simulink model "TVC_Rocket_Model"  (R2025b)
settings: Solver=VariableStepAuto  StartTime=0.0  StopTime=10  RelTol=1e-6
PostLoadFcn:
  | VSS_MODE = 0;
model workspace (MAT data in the model file):
  MMI = 0.012155
  TVC_max = 0.087
  moment_arm = 0.2
  thrust = 14.3
undefined symbols (not defined in the file): Kd, Kp, slew, tau_sensor, theta0
libraries: simulink x1, slpidlib x1, shared3dof x1
settings Model: Creator=joebarnard  LastModifiedBy=braxt
settings SolverCC: ZeroCrossAlgorithm=Adaptive
settings DataIOCC: Refine=5
settings DebuggingCC: IgnoredZcDiagnostic=none  UnconnectedInputMsg=warning  UnconnectedOutputMsg=warning  UnconnectedLineMsg=warning
settings ModelReferenceCC: EnableRefExpFcnMdlSchedulingChecks=on
settings RTWCC: GPUComputeCapability=3.5  DLArmComputeVersion=19.05

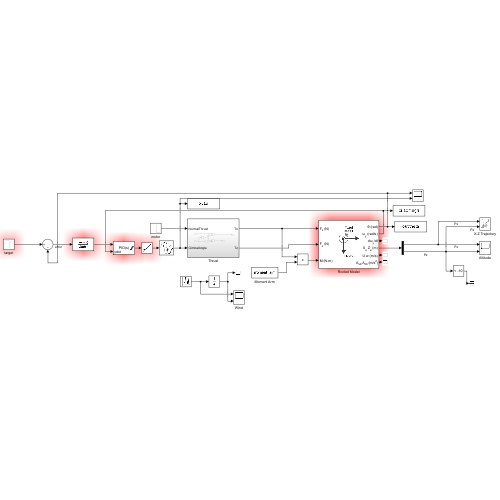
[thumbnail: Simulink's stored preview of the top-level diagram]
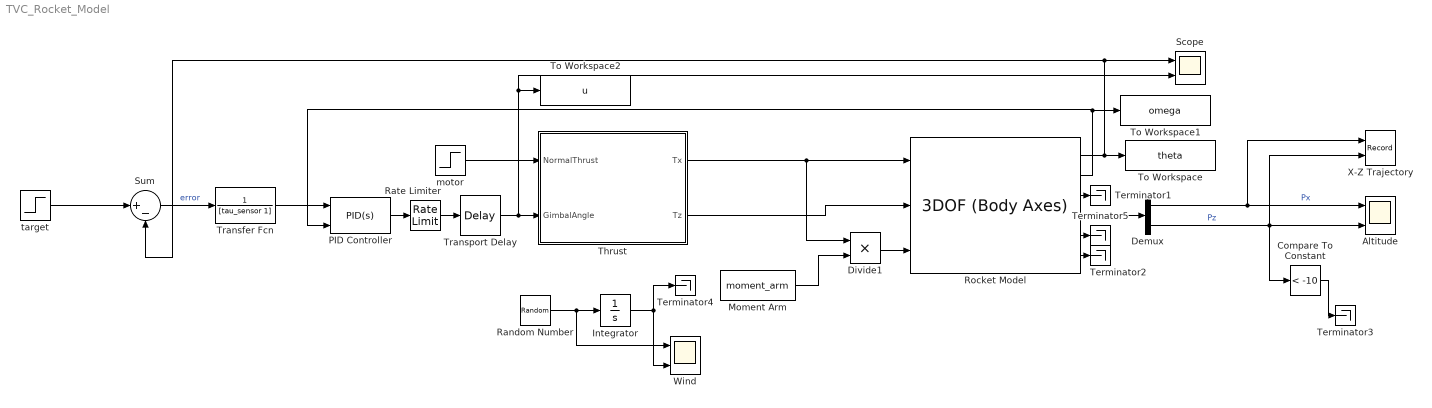
== system TVC_Rocket_Model ==
  Altitude : Scope  NumInputPorts=2
      settings: ActiveDisplayYMinimum=-149.51861  ActiveDisplayYMaximum=1345.66746  DataLoggingVariableName=ScopeData2
  Compare To Constant : simulink/Logic and Bit Operations/Compare To Constant  relop=<  const=-10  OutDataTypeStr=boolean
  Demux : Demux  Outputs=2
  Divide1 : Product  Inputs=**
  Integrator : Integrator
  "Moment Arm " : Constant  Value=moment_arm
  PID Controller : slpidlib/PID Controller  Controller=PID  Form=Parallel  TimeDomain=Continuous-time  UseExternalTs=off  SampleTime=-1  IntegratorMethod=Forward Euler  FilterMethod=Forward Euler  ControllerParametersSource=internal  P=Kp  I=0  UseKiTs=off  D=Kd  UseExternalDerivativeSource=on  N=100  UseFilter=on  TunerSelectOption=Transfer Function Based (PID Tuner App)  InitialConditionSource=internal  InitialConditionForIntegrator=0  InitialConditionForFilter=0  DifferentiatorICPrevScaledInput=0  ExternalReset=none  TrackingMode=off  Kt=1  LimitOutput=on  SatLimitsSource=internal  UpperSaturationLimit=0.087  LowerSaturationLimit=-0.087  LinearizeAsGain=on  AntiWindupMode=none  Kb=1  LimitIntegrator=off  UpperIntegratorSaturationLimit=inf  LowerIntegratorSaturationLimit=-inf  POutMin=[]  POutMax=[]  IOutMin=[]  IOutMax=[]  DOutMin=[]  DOutMax=[]  NOutMin=[]  NOutMax=[]  SumOutMin=[]  SumOutMax=[]  SaturationOutMin=[]  SaturationOutMax=[]  PParamMin=[]  PParamMax=[]  IParamMin=[]  IParamMax=[]  DParamMin=[]  DParamMax=[]  NParamMin=[]  NParamMax=[]  KbParamMin=[]  KbParamMax=[]  KtParamMin=[]  KtParamMax=[]  KbOutMin=[]  KbOutMax=[]  KtOutMin=[]  KtOutMax=[]  IntegratorOutMin=[]  IntegratorOutMax=[]  FilterOutMin=[]  FilterOutMax=[]  SumI1OutMin=[]  SumI1OutMax=[]  SumI2OutMin=[]  SumI2OutMax=[]  SumI3OutMin=[]  SumI3OutMax=[]  SumI4OutMin=[]  SumI4OutMax=[]  SumDOutMin=[]  SumDOutMax=[]  DifferentiatorOutMin=[]  DifferentiatorOutMax=[]  FilterDiffOutCoefMin=[]  FilterDiffOutCoefMax=[]  ReciprocalOutMin=[]  ReciprocalOutMax=[]  SumDenOutMin=[]  SumDenOutMax=[]  SumNumOutMin=[]  SumNumOutMax=[]  DivideOutMin=[]  DivideOutMax=[]  UdiffTsProdOutMin=[]  UdiffTsProdOutMax=[]  NTsProdOutMin=[]  NTsProdOutMax=[]  UintegralTsProdOutMin=[]  UintegralTsProdOutMax=[]  UngainTsProdOutMin=[]  UngainTsProdOutMax=[]  ClampingZeroOutDataTypeStr=Inherit: Inherit via back propagation  ClampingZeroOutMin=[]  ClampingZeroOutMax=[]  FilterDenConstantOutDataTypeStr=Inherit: Inherit via back propagation  FilterDenConstantOutMin=[]  FilterDenConstantOutMax=[]  PCopyOutDataTypeStr=Inherit: Inherit via back propagation  PCopyOutMin=[]  PCopyOutMax=[]  NCopyOutDataTypeStr=Inherit: Inherit via back propagation  NCopyOutMin=[]  NCopyOutMax=[]  IntegratorContinuousStateAttributes=''  IntegratorStateMustResolveToSignalObject=off  IntegratorRTWStateStorageClass=Auto  FilterContinuousStateAttributes=''  FilterStateMustResolveToSignalObject=off  FilterRTWStateStorageClass=Auto  ParallelPVariant=InternalParameters  IdealPVariant=Disabled  IVariant=InternalParameters  DVariant=InternalParameters  IntegratorVariant=Continuous  SatVariant=Enabled  AWVariant=Passthrough  PCopyVariant=Disabled  TRVariant=Disabled  FdbkBlocksVariant=Forward  IdealPFdbkVariant=Disabled  SatFdbkVariant=Disabled  DerivativeFilterVariant=ContFilterOnly  NVariant=InternalParameters  NCopyVariant=Disabled  FilterICVariant=InternalICsFilter  IntegratorICVariant=InternalICs  ExternalResetVariant=Disabled  TRSumVariant=Passthrough  SumFdbkVariant=Disabled  SumVariant=Sum_PID  TsampFilterVariant=InternalTs  TsampNgainVariant=Passthrough  TsampIntegralVariant=Disabled_SignalSpec  ExternalSaturationOutDataTypeStr=Inherit: Same as second input  DerivativeSourceVariant=ExternalYdot  PreIntVariant=InternalPreInt
  Random Number : RandomNumber  Variance=0.0001  Seed=2  SampleTime=3
  Rate Limiter : RateLimiter  RisingSlewLimit=slew  FallingSlewLimit=-slew  SampleTimeMode=inherited
  Rocket Model : shared3dof/3DOF (Body Axes)  units=Metric (MKS)  mtype=Fixed  v_ini=0  theta_ini=theta0  alpha_ini=0  pos_ini=[0 0]  q_ini=0  mass=0.787  mass_e=0.5  mass_f=3.0  Iyy=MMI  Iyy_e=0.5  Iyy_f=3.0  g_in=Internal  g=-9.81  vre_flag=on  abi_flag=off  aMode=0  vel_statename=''  theta_statename=''  pos_statename=''  q_statename=''  mass_statename=''
  Scope : Scope  NumInputPorts=2
      settings: ActiveDisplayYMinimum=-3.9266283739422088  ActiveDisplayYMaximum=3.9256518293177103  DataLoggingVariableName=ScopeData4
  Sum : Sum  Inputs=|+-
  Terminator{1..5} (5 alike) : Terminator
  Thrust : Subsystem
  To Workspace : ToWorkspace  VariableName=theta  SaveFormat=Structure With Time  SampleTime=-1
  To Workspace1 : ToWorkspace  VariableName=omega  SaveFormat=Structure With Time  SampleTime=-1
  To Workspace2 : ToWorkspace  VariableName=u  SaveFormat=Structure With Time  SampleTime=-1
  Transfer Fcn : TransferFcn  Denominator=[tau_sensor 1]
  Transport Delay : TransportDelay  DelayTime=0
  Wind : Scope  NumInputPorts=2
      settings: ActiveDisplayYMinimum=-0.02114  ActiveDisplayYMaximum=0.01688
  X-Z Trajectory : Record  NumPorts=2.0  FileSettingsInternal="{\"entries\":[{\"content\":{\"excelSettings\":{\"content\":{},\"type\":\"Streamout.ExcelSettings\"},\"parquetSettings\":{\"content\":{},\"type\":\"Streamout.ParquetSettings\"}},\"type\":\"Streamout.FileSettingStorage\",\"uuid\":\"\"}],\"packageUris\":[\"http:\\/\\/schema.mathworks.com\\/mf0\\/streamout_blocks\\/R2020a\"],\"version\":\"1.0\"}"  FrameSettings=[0, 0]  Layout=[1 1]  SignalsInternal="{\"entries\":[{\"content\":{\"signals\":[{\"content\":{\"blockPath\":[],\"dimensions\":[1],\"domain\":\"\",\"lineColor\":\"#a2142f\",\"plots\":[ 1 ],\"port\":1,\"signalID\":1,\"signalName\":\"Px\"},\"type\":\"RecordBlkView.Signal\",\"uuid\":\"\"},{\"content\":{\"blockPath\":[],\"dimensions\":[1],\"domain\":\"\",\"lineColor\":\"#139fff\",\"plots\":[ 1 ],\"port\":2,\"signalID\":2,\"signalName\":\"Pz\"},\"type\":\"RecordBlkView.Signal\",\"uuid\":\"\"}]},\"type\":\"RecordBlkView.InputSignals\",\"uuid\":\"\"}],\"packageUris\":[\"http:\\/\\/schema.mathworks.com\\/mf0\\/streamout_blocks\\/R2020a\"],\"version\":\"1.0\"}"  VisualizationBindings="{\"xyplotplugin\":{\"info\":[{\"series\":[{\"bindingParametersList\":[{\"parameter\":\"X-Axis\",\"signalID\":1,\"signalName\":\"Px\"},{\"parameter\":\"Y-Axis\",\"signalID\":2,\"signalName\":\"Pz\"}],\"seriesID\":0}],\"subplotID\":1}]}}"  CompatibilityTag=XY  st=-1
  motor : Step  Time=20  Before=thrust  After=0  SampleTime=0
  target : Step  Before=theta0  After=0  SampleTime=0
  wires:
  Rocket Model/4 -> Demux/1
  motor/1 -> Thrust/1(NormalThrust)
  Thrust/1(Tx) -> Rocket Model/1, Divide1/1
  Thrust/2(Tz) -> Rocket Model/2
  "Moment Arm "/1 -> Divide1/2
  Random Number/1 -> Wind/1, Integrator/1
  Integrator/1 -> Terminator4/1, Wind/2
  Divide1/1 -> Rocket Model/3
  Demux/2 -> Altitude/2, Compare To Constant/1, X-Z Trajectory/2  "Pz"
  Demux/1 -> X-Z Trajectory/1, Altitude/1  "Px"
  Compare To Constant/1 -> Terminator3/1
  Rocket Model/1 -> To Workspace/1, Sum/2, Scope/1
  Rocket Model/2 -> To Workspace1/1, PID Controller/2
  PID Controller/1 -> Rate Limiter/1
  Rocket Model/6 -> Terminator2/1
  Rocket Model/3 -> Terminator1/1
  target/1 -> Sum/1
  Sum/1 -> Transfer Fcn/1  "error"
  Rate Limiter/1 -> Transport Delay/1
  Transport Delay/1 -> To Workspace2/1, Scope/2, Thrust/2(GimbalAngle)
  Rocket Model/5 -> Terminator5/1
  Transfer Fcn/1 -> PID Controller/1

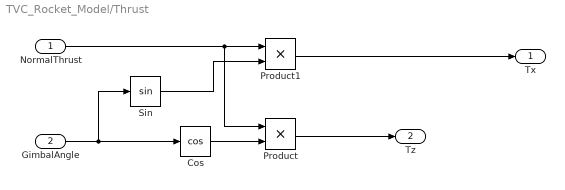
== system TVC_Rocket_Model/Thrust ==
  NormalThrust : Inport
  GimbalAngle : Inport  Port=2
  Cos : Trigonometry  Operator=cos
  Product : Product  RndMeth=Zero
  Product1 : Product  RndMeth=Zero
  Sin : Trigonometry
  Tx : Outport
  Tz : Outport  Port=2
  wires:
  GimbalAngle/1 -> Cos/1, Sin/1
  Product/1 -> Tz/1
  Cos/1 -> Product/2
  NormalThrust/1 -> Product/1, Product1/1
  Sin/1 -> Product1/2
  Product1/1 -> Tx/1
